simulink model "Transf_3f1"  (Simulink 4.00)
settings: Solver=ode23tb  StartTime=0.0  StopTime=0.1
libraries: powerlib2 x3, powerlib_extras x2
settings Model: BlockReductionOpt=off

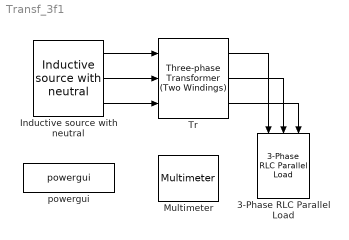
== system Transf_3f1 ==
  3-Phase RLC Parallel Load : powerlib_extras/Three-Phase Library/3-Phase RLC Parallel Load  Orientation=down  Vpp=380  fn=50  P3=100e3  QL3=50e3  QC3=0
  Inductive source with neutral : powerlib_extras/Three-Phase Library/Inductive source with neutral  V=1000  Phi=0  F=50  R=0.001  L=1e-4
  Multimeter : powerlib2/Measurements/Multimeter  Tag=PoWeRsYsTeMmEaSuReMeNt  sel=[1 7 13]  L=15  Gain=[1 1 1]  yselected=[411,8.0002441406250000e+000;441,8.0002441406250000e+000;570,8.0002441406250000e+000]  PSBOutputType=1  PSBequivalent=1  AxesSetting=[0,0.1,-100,100]  Display=1  SavedBlockNames=-11
  Tr : powerlib2/Elements/Three-phase Transformer (Two Windings)  Tag=PoWeRsYsTeMbLoCk  nominal=[ 500e3 , 50 ]  type1=Y  params1=[ 660 , 0.02 , 0.8 ]  type2=Y  params2=[ 380 , 0.02 , 0.8 ]  ynsat=off  rmag=500  lm=500  sat="[ 0,0  ;  0.005,1.2  ;  1.0,1.4 ]"  sif=off  phi0=[ 0.8 , -0.8 , 0.7 ]  mesure=All measurements (V I Fluxes)  PSBOutputType=1111
  powergui : powerlib2/powergui  matfilesaved=off  Frange=logspace(0,3,50)  Ylog=off  Xlog=off  save=off  variable=ZData  display=off
  wires:
  Inductive source with neutral/1 -> Tr/1
  Inductive source with neutral/2 -> Tr/2
  Inductive source with neutral/3 -> Tr/3
  Tr/1 -> 3-Phase RLC Parallel Load/1
  Tr/2 -> 3-Phase RLC Parallel Load/2
  Tr/3 -> 3-Phase RLC Parallel Load/3
